simulink model "tuned_mass_damper_BLOCK"  (R2024a)
settings: Solver=ode4  StartTime=0.0  StopTime=180.0  FixedStep=0.02  RelTol=1e-3
values from neighbouring files (symbols this model uses):
  c1 = 1887.4    [tuned_mass_damper.m]
  c2 = 59.8026    [tuned_mass_damper.m]
  F_frq = 0.8954    [tuned_mass_damper.m]
  F_mag = 200    [tuned_mass_damper.m]
  k1 = 42250    [tuned_mass_damper.m]
  k2 = 526.6805    [tuned_mass_damper.m]
  m1 = 52696    [tuned_mass_damper.m]
  m2 = 658.7    [tuned_mass_damper.m]
settings Model: Creator=Onurcan Okay  LastModifiedBy=Onurcan Okay

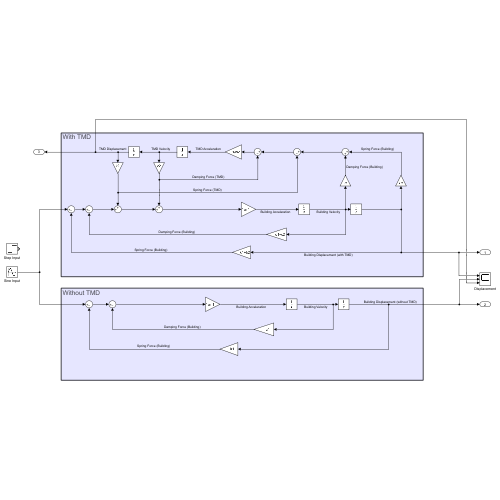
[thumbnail: Simulink's stored preview of the top-level diagram]
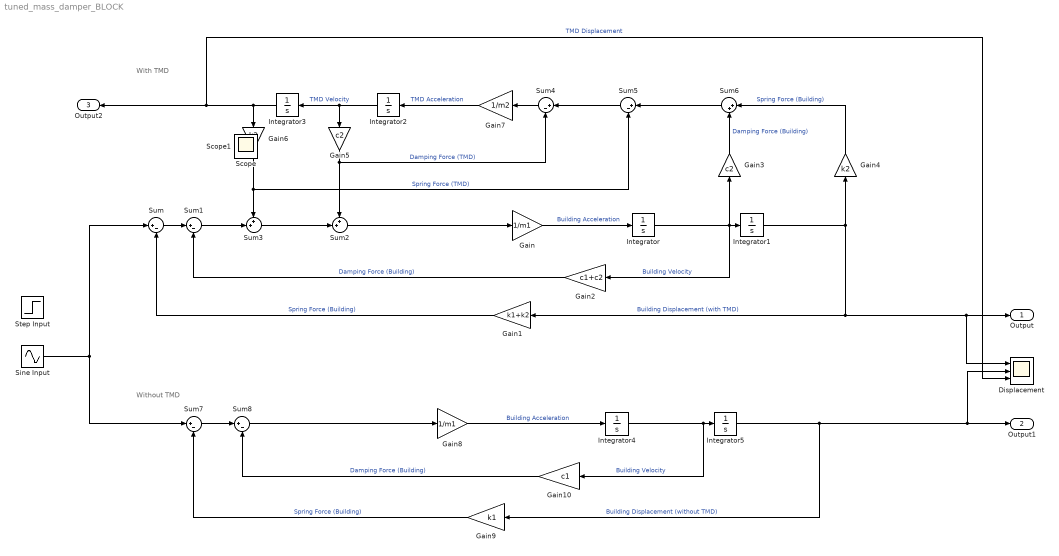
== system tuned_mass_damper_BLOCK ==
  note: With TMD
  note: Without TMD
  Displacement : Scope  NumInputPorts=3
  Gain : Gain  Gain=1/m1
  Gain1 : Gain  Gain=k1+k2
  Gain10 : Gain  Gain=c1
  Gain2 : Gain  Gain=c1+c2
  Gain3 : Gain  Gain=c2
  Gain4 : Gain  Gain=k2
  Gain5 : Gain  Gain=c2
  Gain6 : Gain  Gain=k2
  Gain7 : Gain  Gain=1/m2
  Gain8 : Gain  Gain=1/m1
  Gain9 : Gain  Gain=k1
  Integrator{,1..5} (6 alike) : Integrator
  Sine Input : Sin  Amplitude=F_mag  Frequency=F_frq  SampleTime=0
  Step Input : Step  SampleTime=0
  Sum{,1,4..5,7..8} (6 alike) : Sum  Inputs=|+-
  Sum2 : Sum  Inputs=++|
  Sum3 : Sum  Inputs=++|
  Sum6 : Sum  Inputs=|++
  Output : Outport
  Output1 : Outport  Port=2
  Output2 : Outport  Port=3
  Scope : Scope
  Scope1 : Scope
  wires:
  Sum7/1 -> Sum8/1
  Integrator5/1 -> Output1/1, Displacement/2, Gain9/1  "Building Displacement (without TMD)"
  Integrator4/1 -> Gain10/1, Integrator5/1  "Building Velocity"
  Sum8/1 -> Gain8/1
  Gain10/1 -> Sum8/2  "Damping Force (Building)"
  Gain8/1 -> Integrator4/1  "Building Acceleration"
  Gain9/1 -> Sum7/2  "Spring Force (Building)"
  Gain4/1 -> Sum6/1  "Spring Force (Building)"
  Sum3/1 -> Sum2/2
  Gain1/1 -> Sum/2  "Spring Force (Building)"
  Sum6/1 -> Sum5/1
  Gain7/1 -> Integrator2/1  "TMD Acceleration"
  Gain2/1 -> Sum1/2  "Damping Force (Building)"
  Gain/1 -> Integrator/1  "Building Acceleration"
  Sum4/1 -> Gain7/1
  Gain3/1 -> Sum6/2  "Damping Force (Building)"
  Sum5/1 -> Sum4/1
  Sum2/1 -> Gain/1
  Integrator/1 -> Gain3/1, Gain2/1, Integrator1/1  "Building Velocity"
  Integrator3/1 -> Output2/1, Displacement/3, Gain6/1  "TMD Displacement"
  Sum1/1 -> Sum3/2
  Sum/1 -> Sum1/1
  Integrator2/1 -> Integrator3/1, Gain5/1  "TMD Velocity"
  Gain6/1 -> Sum5/2, Sum3/1  "Spring Force (TMD)"
  Integrator1/1 -> Output/1, Displacement/1, Gain1/1, Gain4/1  "Building Displacement (with TMD)"
  Gain5/1 -> Sum2/1, Sum4/2  "Damping Force (TMD)"
  Sine Input/1 -> Sum7/1, Sum/1
